simulink model "komparacija"  (R2020a)
settings: Solver=ode5  StartTime=0.0  StopTime=tfin  FixedStep=1e-3  RelTol=1e-3
values from neighbouring files (symbols this model uses):
  beta = S_upper_limit*w0/2    (= 0.06550194)    [komparacija_matlab.m]
  derivative_e_lower_limit = -7.8663    [komparacija_matlab.m]
  derivative_e_upper_limit = 7.8663    [komparacija_matlab.m]
  disturb_X = 0.2*Xe    (= 0.978133730754)    [komparacija_matlab.m]
  disturb_X_time = 5    [komparacija_matlab.m]
  F_lower_limit = 0    [komparacija_matlab.m]
  F_upper_limit = Fe + 1e-3*Fe    (= 3.21211951185)    [komparacija_matlab.m]
  F_upper_limit_PI = 1e-3*Fe    (= 0.00320891060125)    [komparacija_matlab.m]
  Fe = 3.20891060125344    (= 3.20891060125)    [komparacija_matlab.m]
  Fi = beta/5/w0    (= 0.02324)    [komparacija_matlab.m]
  K0_FLRT = w0    (= 0.5637)    [komparacija_matlab.m]
  K1 = 0.0300    (= 0.03)    [komparacija_matlab.m]
  K2 = 0.5000    (= 0.5)    [komparacija_matlab.m]
  Kc1 = 1/abs(freqresp((1+1/Ti1/s)*G_design,w1_design))    [komparacija_matlab.m]
  Ki = 0    [komparacija_matlab.m]
  mi0 = mie    (= 0.802227650313)    [komparacija_matlab.m]
  mi_max = 1    [komparacija_matlab.m]
  S_step1 = delta    (= 0)    [komparacija_matlab.m]
  S_step2 = delta    (= 0)    [komparacija_matlab.m]
  S_time_step1 = 20    [komparacija_matlab.m]
  S_time_step2 = 50    [komparacija_matlab.m]
  Se = 0.218662692463450    (= 0.218662692463)    [komparacija_matlab.m]
  SF = 10.0000    (= 10)    [komparacija_matlab.m]
  std_noise = 1e-5*Se    (= 2.18662692463e-06)    [komparacija_matlab.m]
  V = 4.0000    (= 4)    [komparacija_matlab.m]
  x10 = Xe    (= 4.89066865377)    [komparacija_matlab.m]
  x20 = Se    (= 0.218662692463)    [komparacija_matlab.m]
  Y = 0.5000    (= 0.5)    [komparacija_matlab.m]
undefined symbols (not defined in the file or in its folder): magnitude
libraries: fuzblock x1, cstblocks x1
settings Model: Creator=anaMceranic  LastModifiedBy=anaMceranic
settings DataIOCC: ReturnWorkspaceOutputs=off

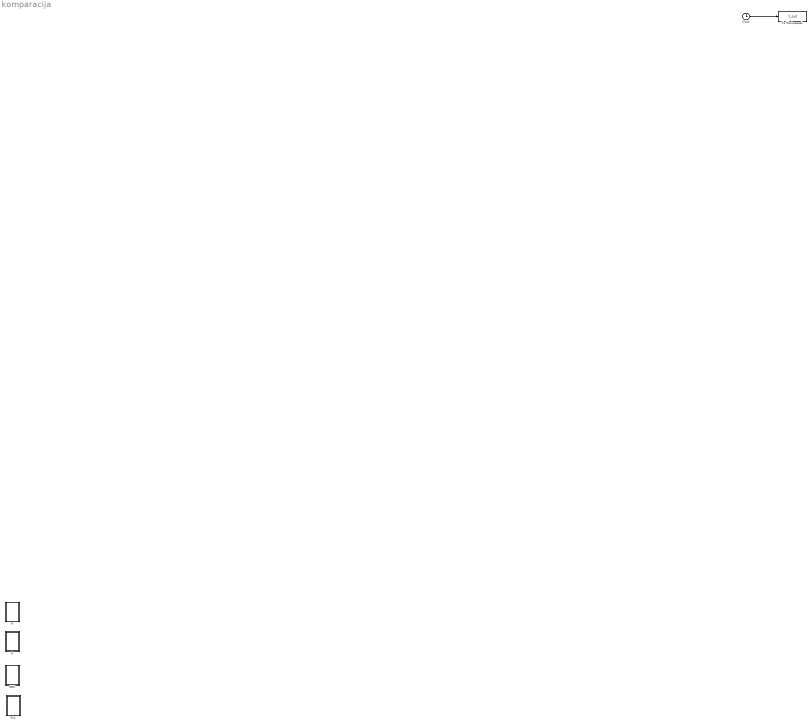
== system komparacija ==
  Clock : Clock
  FLC : Subsystem
  PI : Subsystem
  SMC : Subsystem
  To Workspace1 : ToWorkspace  VariableName=t_out  SampleTime=-1
  fl : Subsystem
  wires:
  Clock/1 -> To Workspace1/1

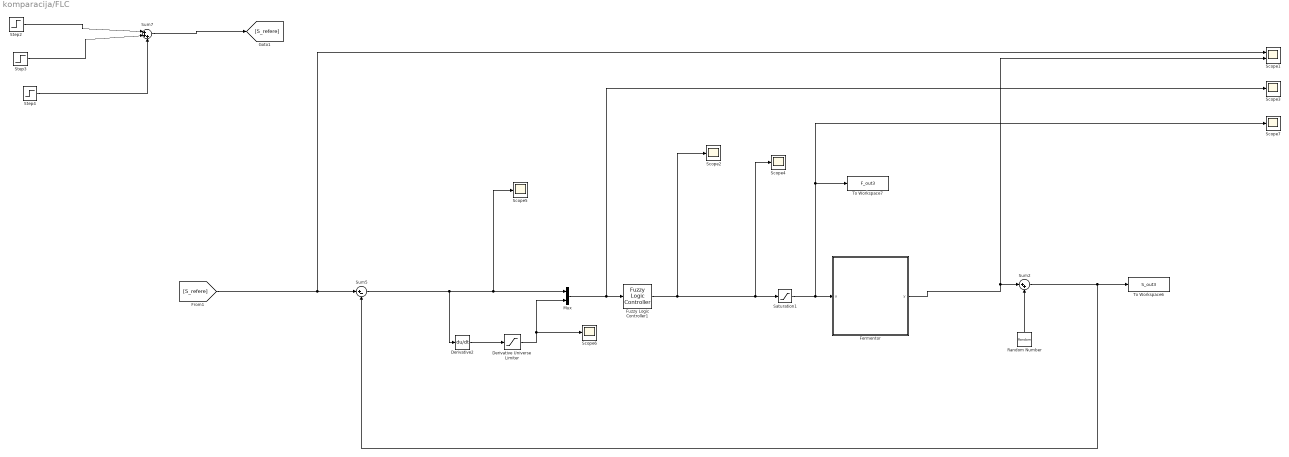
== system komparacija/FLC ==
  Derivative Universe Limiter : Saturate  UpperLimit=derivative_e_upper_limit  LowerLimit=derivative_e_lower_limit
  Derivative2 : Derivative
  Fermentor : Subsystem
  Fuzzy Logic Controller1 : fuzblock/Fuzzy Logic  Controller  FIS=FLC  OutputSampleNumber=101  DataType=double  FuzzifiedInputs=off  RuleFiringStrengths=off  RuleOutputs=off  AggregatedOutputs=off  SimulateUsing=Interpreted execution  OutOfRangeInputValueMessage=warning  NoRuleFiredMessage=warning  EmptyOutputFuzzySetMessage=warning
  Mux : Mux  Inputs=2
  Random Number : RandomNumber  Variance=std_noise  SampleTime=0.1
  Saturation1 : Saturate  UpperLimit=F_upper_limit  LowerLimit=F_lower_limit
  Scope1 : Scope  NumInputPorts=2
  Scope{2..7} (6 alike) : Scope
  Step2 : Step  Time=0  Before=Se  After=Se  SampleTime=0
  Step3 : Step  Time=S_time_step1  After=S_step1  SampleTime=0
  Step4 : Step  Time=S_time_step2  After=-S_step2  SampleTime=0
  Sum2 : Sum  Inputs=|++
  Sum5 : Sum  Inputs=|+-
  Sum7 : Sum  Inputs=|+++
  To Workspace6 : ToWorkspace  VariableName=S_out3  SampleTime=-1
  To Workspace7 : ToWorkspace  VariableName=F_out3  SampleTime=-1
  wires:
  Fuzzy Logic Controller1/1 -> Scope4/1, Saturation1/1, Scope2/1
  Sum5/1 -> Derivative2/1, Scope5/1, Mux/1
  [S_refere] -> Scope1/1, Sum5/1
  Fermentor/1(y) -> Scope1/2, Sum2/1
  Sum2/1 -> Sum5/2, To Workspace6/1
  Step2/1 -> Sum7/1
  Saturation1/1 -> Scope7/1, To Workspace7/1, Fermentor/1(u)
  Random Number/1 -> Sum2/2
  Derivative Universe Limiter/1 -> Scope6/1, Mux/2
  Mux/1 -> Fuzzy Logic Controller1/1, Scope3/1
  Step3/1 -> Sum7/2
  Sum7/1 -> [S_refere]
  Derivative2/1 -> Derivative Universe Limiter/1
  Step4/1 -> Sum7/3

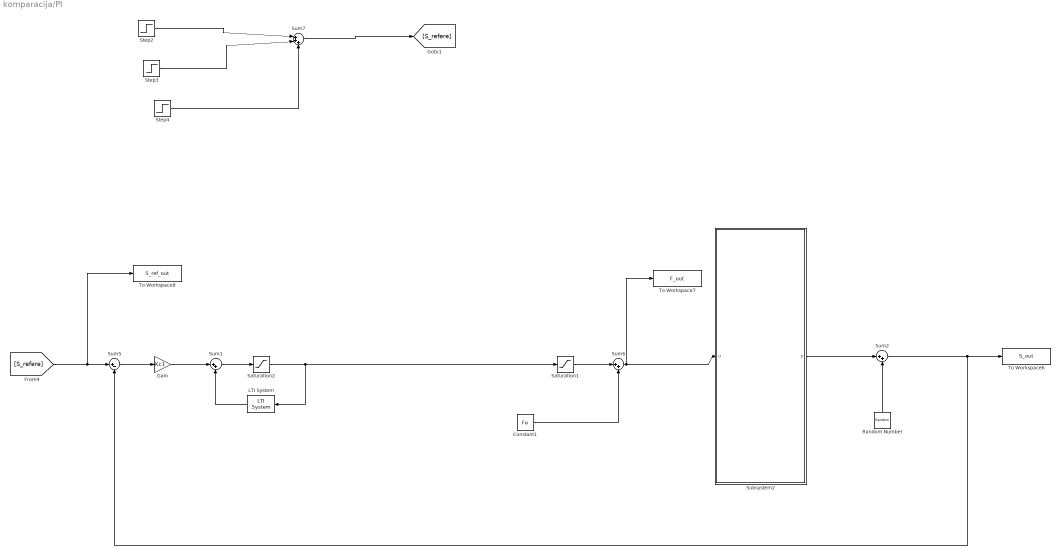
== system komparacija/PI ==
  Constant1 : Constant  Value=Fe
  Gain : Gain  Gain=Kc1
  LTI System : cstblocks/LTI System  sys=KPI_aw  IC=[]
  Random Number : RandomNumber  Variance=std_noise  SampleTime=0.1
  Saturation1 : Saturate  UpperLimit=F_upper_limit_PI  LowerLimit=F_lower_limit
  Saturation2 : Saturate  UpperLimit=F_upper_limit  LowerLimit=F_lower_limit
  Step2 : Step  Time=0  Before=Se  After=Se  SampleTime=0
  Step3 : Step  Time=S_time_step1  After=S_step1  SampleTime=0
  Step4 : Step  Time=S_time_step2  After=-S_step2  SampleTime=0
  Subsystem2 : Subsystem
  Sum1 : Sum  Inputs=|++
  Sum2 : Sum  Inputs=|++
  Sum5 : Sum  Inputs=|+-
  Sum6 : Sum  Inputs=|++
  Sum7 : Sum  Inputs=|+++
  To Workspace6 : ToWorkspace  VariableName=S_out  SampleTime=-1
  To Workspace7 : ToWorkspace  VariableName=F_out  SampleTime=-1
  To Workspace8 : ToWorkspace  VariableName=S_ref_out  SampleTime=-1
  wires:
  [S_refere] -> To Workspace8/1, Sum5/1
  Sum5/1 -> Gain/1
  Saturation2/1 -> Saturation1/1, LTI System/1
  Sum6/1 -> To Workspace7/1, Subsystem2/1(u)
  Sum1/1 -> Saturation2/1
  Sum7/1 -> [S_refere]
  Constant1/1 -> Sum6/2
  Subsystem2/1(y) -> Sum2/1
  Gain/1 -> Sum1/1
  Step2/1 -> Sum7/1
  Saturation1/1 -> Sum6/1
  Step4/1 -> Sum7/3
  Step3/1 -> Sum7/2
  Sum2/1 -> Sum5/2, To Workspace6/1
  Random Number/1 -> Sum2/2
  LTI System/1 -> Sum1/2

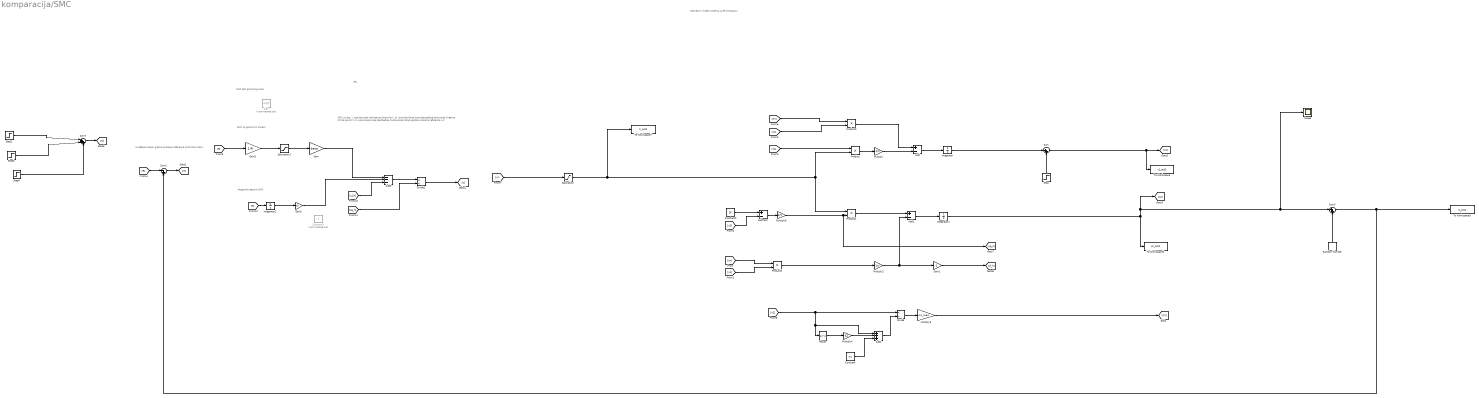
== system komparacija/SMC ==
  note: SMC bez graničnog sloja
  note: eFL
  note: integralno dejstvo SMC
  note: SMC skupa:
      | 1. poništavanje nelinearne dinamike
      | 2. a) upravljavljanje koje obezbeđuje dostizanje linearne klizne površi
      | 2. b) upravljanje koje obezbeđuje zavšavanje stanja greške praćenja reference u 0
  note: Nelinearni model sistema za fermentaciju
  note: SMC sa graničnim slojem
  note: Uvođenje stanja:
      | greška praćenja reference od strane izlaza
  Add : Sum  Inputs=+-
  Add1 : Sum  Inputs=+-
  Add2 : Sum  Inputs=+++
  Add3 : Sum  Inputs=---
  Constant : Constant  Value=K1
  Constant1 : Constant  Commented=on  Value=0
  Constant2 : Constant  Value=SF
  Divide : Product  Inputs=*/
  Divide1 : Product  Inputs=*/
  Gain : Gain  Gain=beta
  Gain1 : Gain  Gain=-1
  Gain2 : Gain  Gain=Ki
  Gain3 : Gain  Gain=1/Fi
  Integrator : Integrator  InitialCondition=x10
  Integrator1 : Integrator  InitialCondition=x20
  Integrator2 : Integrator
  Multiply : Gain  Gain=1/V
  Multiply2 : Gain  Gain=1/Y
  Multiply3 : Gain  Gain=mi_max
  Multiply4 : Gain  Gain=K2
  Multiply6 : Gain  Gain=1/V
  Power : Math  Operator=magnitude^2  SaturateOnIntegerOverflow=on
  Product{,1..3} (4 alike) : Product
  Random Number : RandomNumber  Variance=std_noise  SampleTime=0.1
  Saturation : Saturate  UpperLimit=F_upper_limit  LowerLimit=F_lower_limit
  Saturation1 : Saturate
  Scope : Scope
  Sign : Signum  Commented=on
  Step : Step  Time=disturb_X_time  After=disturb_X  SampleTime=0
  Step2 : Step  Time=0  Before=Se  After=Se  SampleTime=0
  Step3 : Step  Time=S_time_step1  After=S_step1  SampleTime=0
  Step4 : Step  Time=S_time_step2  After=-S_step2  SampleTime=0
  Subtract : Sum  Inputs=+-
  Sum : Sum  Inputs=|++
  Sum2 : Sum  Inputs=|-+
  Sum3 : Sum  Inputs=|++
  Sum7 : Sum  Inputs=|+++
  To Workspace : ToWorkspace  VariableName=x1_out2  SampleTime=-1
  To Workspace2 : ToWorkspace  VariableName=x2_out2  SampleTime=-1
  To Workspace3 : ToWorkspace  VariableName=S_out2  SampleTime=-1
  To Workspace7 : ToWorkspace  VariableName=F_out2  SampleTime=-1
  wires:
  Step/1 -> Sum/2
  Integrator/1 -> Sum/1
  [mi] -> Product3/1
  [mi] -> Product2/1
  [e] -> Gain3/1
  Product3/1 -> Add/1
  Subtract/1 -> Multiply6/1
  Sum3/1 -> Sum2/2, To Workspace3/1
  Multiply3/1 -> [mi]
  Saturation/1 -> To Workspace7/1, Product1/1, Product/2
  Gain3/1 -> Saturation1/1
  Saturation1/1 -> Gain/1
  Add3/1 -> Divide1/1
  Constant2/1 -> Subtract/1
  [Lf_h] -> Add3/3
  Integrator1/1 -> Scope/1, Sum3/1, [x2], To Workspace2/1
  Multiply2/1 -> Gain1/1, Add1/2
  Constant/1 -> Add2/3
  Product2/1 -> Multiply2/1
  [x1] -> Product/1
  Sum7/1 -> [R]
  Multiply4/1 -> Add2/2
  Product/1 -> Multiply/1
  Step3/1 -> Sum7/2
  Add2/1 -> Divide/2
  [x2] -> Subtract/2
  [u] -> Saturation/1
  Gain/1 -> Add3/1
  Add/1 -> Integrator/1
  Step2/1 -> Sum7/1
  Integrator2/1 -> Gain2/1
  Multiply6/1 -> [Lg_h], Product1/2
  Divide/1 -> Multiply3/1
  Gain2/1 -> Add3/2
  Gain1/1 -> [Lf_h]
  [x1] -> Product3/2
  [e] -> Integrator2/1
  [R] -> Sum2/1
  Sum2/1 -> [e]
  [Lg_h] -> Divide1/2
  Random Number/1 -> Sum3/2
  Divide1/1 -> [u]
  Product1/1 -> Add1/1
  [x1] -> Product2/2
  Add1/1 -> Integrator1/1
  Sum/1 -> [x1], To Workspace/1
  Multiply/1 -> Add/2
  Step4/1 -> Sum7/3
  [x2] -> Power/1, Add2/1, Divide/1
  Power/1 -> Multiply4/1

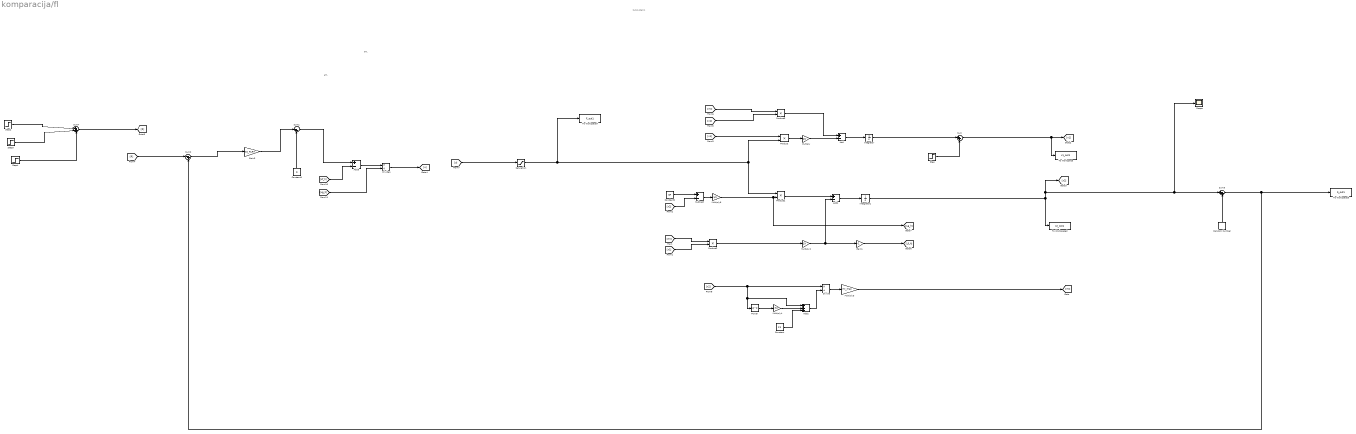
== system komparacija/fl ==
  note: eFL
  note: Subsystem1
  note: eFL
  Add : Sum  Inputs=+-
  Add1 : Sum  Inputs=+-
  Add2 : Sum  Inputs=+++
  Add3 : Sum  Inputs=+-
  Constant : Constant  Value=K1
  Constant1 : Constant  Value=0
  Constant2 : Constant  Value=SF
  Divide : Product  Inputs=*/
  Divide1 : Product  Inputs=*/
  Gain1 : Gain  Gain=-1
  Gain3 : Gain  Gain=K0_FLRT
  Integrator : Integrator  InitialCondition=x10
  Integrator1 : Integrator  InitialCondition=x20
  Multiply : Gain  Gain=1/V
  Multiply2 : Gain  Gain=1/Y
  Multiply3 : Gain  Gain=mi_max
  Multiply4 : Gain  Gain=K2
  Multiply6 : Gain  Gain=1/V
  Power : Math  Operator=magnitude^2  SaturateOnIntegerOverflow=on
  Product{,1..3} (4 alike) : Product
  Random Number : RandomNumber  Variance=std_noise  SampleTime=0.1
  Saturation : Saturate  UpperLimit=F_upper_limit  LowerLimit=F_lower_limit
  Scope : Scope
  Step : Step  Time=5  After=disturb_X  SampleTime=0
  Step2 : Step  Time=0  Before=Se  After=Se  SampleTime=0
  Step3 : Step  Time=S_time_step1  After=S_step1  SampleTime=0
  Step4 : Step  Time=S_time_step2  After=-S_step2  SampleTime=0
  Subtract : Sum  Inputs=+-
  Sum : Sum  Inputs=|++
  Sum1 : Sum  Inputs=|--
  Sum2 : Sum  Inputs=|-+
  Sum3 : Sum  Inputs=|++
  Sum7 : Sum  Inputs=|+++
  To Workspace : ToWorkspace  VariableName=x1_out1  SampleTime=-1
  To Workspace2 : ToWorkspace  VariableName=x2_out1  SampleTime=-1
  To Workspace3 : ToWorkspace  VariableName=S_out1  SampleTime=-1
  To Workspace7 : ToWorkspace  VariableName=F_out1  SampleTime=-1
  wires:
  Saturation/1 -> To Workspace7/1, Product1/1, Product/2
  [x2] -> Power/1, Add2/1, Divide/1
  [x2] -> Subtract/2
  Product3/1 -> Add/1
  [mi] -> Product2/1
  Integrator1/1 -> Scope/1, Sum3/1, [x2], To Workspace2/1
  Sum3/1 -> Sum2/2, To Workspace3/1
  Constant1/1 -> Sum1/2
  Step4/1 -> Sum7/3
  Subtract/1 -> Multiply6/1
  [x1] -> Product/1
  Sum7/1 -> [R]
  Step/1 -> Sum/2
  Multiply4/1 -> Add2/2
  [x1] -> Product3/2
  Gain3/1 -> Sum1/1
  Add3/1 -> Divide1/1
  Sum1/1 -> Add3/1
  Multiply3/1 -> [mi]
  [R] -> Sum2/1
  Sum2/1 -> Gain3/1
  Add2/1 -> Divide/2
  Product/1 -> Multiply/1
  Add1/1 -> Integrator1/1
  [u] -> Saturation/1
  Constant/1 -> Add2/3
  Multiply/1 -> Add/2
  Product1/1 -> Add1/1
  Power/1 -> Multiply4/1
  Multiply2/1 -> Gain1/1, Add1/2
  Multiply6/1 -> [Lg_h], Product1/2
  Divide1/1 -> [u]
  [Lf_h] -> Add3/2
  Divide/1 -> Multiply3/1
  Gain1/1 -> [Lf_h]
  Add/1 -> Integrator/1
  Integrator/1 -> Sum/1
  Constant2/1 -> Subtract/1
  Product2/1 -> Multiply2/1
  Sum/1 -> [x1], To Workspace/1
  Step3/1 -> Sum7/2
  [x1] -> Product2/2
  [Lg_h] -> Divide1/2
  [mi] -> Product3/1
  Random Number/1 -> Sum3/2
  Step2/1 -> Sum7/1

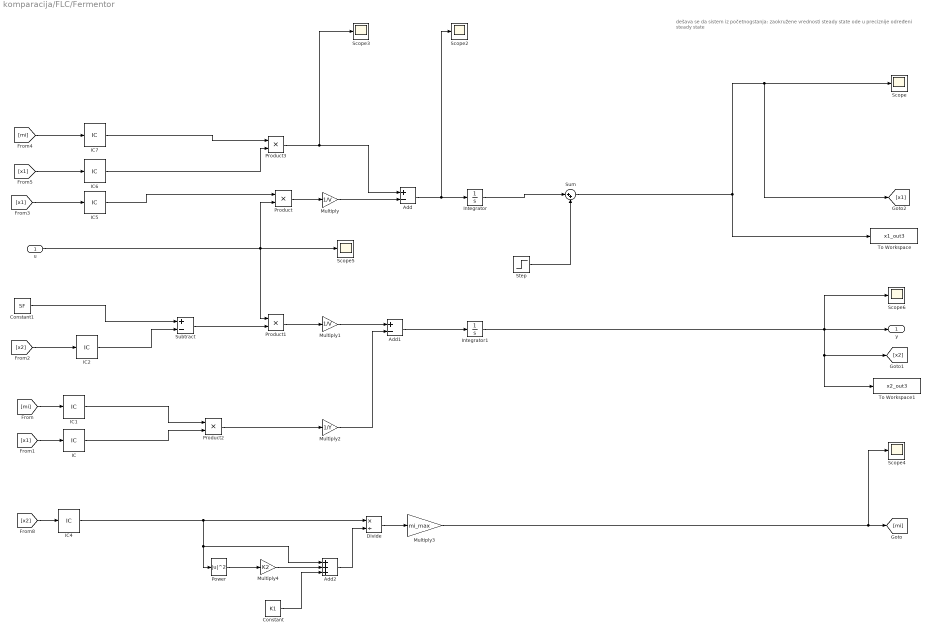
== system komparacija/FLC/Fermentor ==
  note: dešava se da sistem iz početnogstanja: zaokružene vrednosti steady state
      | ode u preciznije određeni steady state
  u : Inport
  Add : Sum  Inputs=+-
  Add1 : Sum  Inputs=+-
  Add2 : Sum  Inputs=+++
  Constant : Constant  Value=K1
  Constant1 : Constant  Value=SF
  Divide : Product  Inputs=*/
  IC : InitialCondition  Value=x10
  IC1 : InitialCondition  Value=mi0
  IC2 : InitialCondition  Value=x20
  IC4 : InitialCondition  Value=x20
  IC5 : InitialCondition  Value=x10
  IC6 : InitialCondition  Value=x10
  IC7 : InitialCondition  Value=mi0
  Integrator : Integrator  InitialCondition=x10
  Integrator1 : Integrator  InitialCondition=x20
  Multiply : Gain  Gain=1/V
  Multiply1 : Gain  Gain=1/V
  Multiply2 : Gain  Gain=1/Y
  Multiply3 : Gain  Gain=mi_max
  Multiply4 : Gain  Gain=K2
  Power : Math  Operator=magnitude^2  SaturateOnIntegerOverflow=on
  Product{,1..3} (4 alike) : Product
  Scope{,2..6} (6 alike) : Scope
  Step : Step  Time=disturb_X_time  After=disturb_X  SampleTime=0
  Subtract : Sum  Inputs=+-
  Sum : Sum  Inputs=|++
  To Workspace : ToWorkspace  VariableName=x1_out3  SampleTime=-1
  To Workspace1 : ToWorkspace  VariableName=x2_out3  SampleTime=-1
  y : Outport
  wires:
  [x1] -> IC/1
  Product2/1 -> Multiply2/1
  Multiply/1 -> Add/2
  Add2/1 -> Divide/2
  Constant/1 -> Add2/3
  [x1] -> IC6/1
  Multiply4/1 -> Add2/2
  [mi] -> IC1/1
  Power/1 -> Multiply4/1
  [x2] -> IC2/1
  Add1/1 -> Integrator1/1
  Multiply2/1 -> Add1/2
  Divide/1 -> Multiply3/1
  Product3/1 -> Scope3/1, Add/1
  u/1 -> Product/2, Product1/1, Scope5/1
  [x1] -> IC5/1
  Multiply1/1 -> Add1/1
  Product1/1 -> Multiply1/1
  Subtract/1 -> Product1/2
  [x2] -> IC4/1
  Add/1 -> Scope2/1, Integrator/1
  Product/1 -> Multiply/1
  [mi] -> IC7/1
  Multiply3/1 -> [mi], Scope4/1
  Integrator1/1 -> Scope6/1, To Workspace1/1, [x2], y/1
  IC/1 -> Product2/2
  IC1/1 -> Product2/1
  IC2/1 -> Subtract/2
  Constant1/1 -> Subtract/1
  IC4/1 -> Divide/1, Add2/1, Power/1
  IC5/1 -> Product/1
  IC6/1 -> Product3/2
  IC7/1 -> Product3/1
  Sum/1 -> To Workspace/1, Scope/1, [x1]
  Step/1 -> Sum/2
  Integrator/1 -> Sum/1

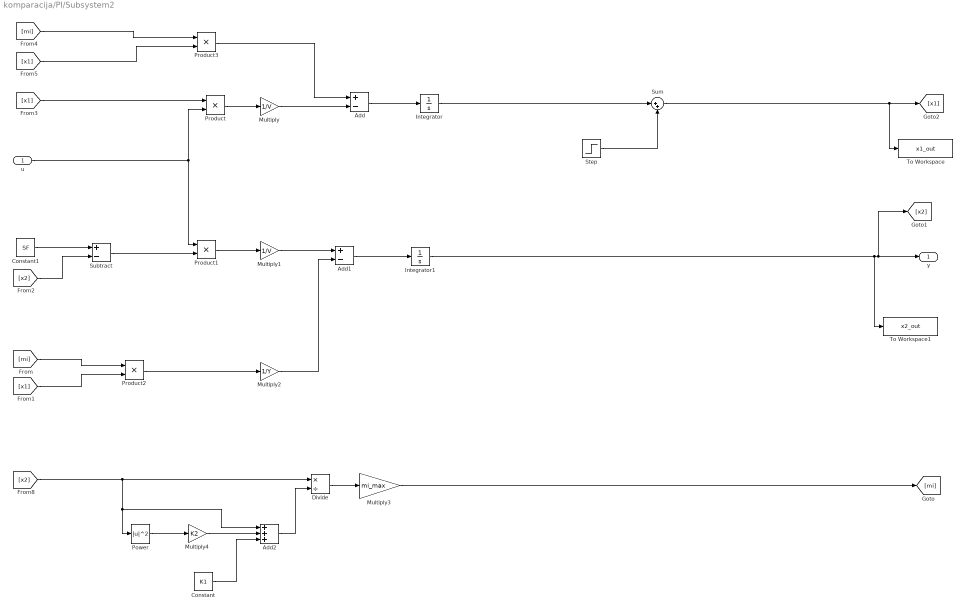
== system komparacija/PI/Subsystem2 ==
  u : Inport
  Add : Sum  Inputs=+-
  Add1 : Sum  Inputs=+-
  Add2 : Sum  Inputs=+++
  Constant : Constant  Value=K1
  Constant1 : Constant  Value=SF
  Divide : Product  Inputs=*/
  Integrator : Integrator  InitialCondition=x10
  Integrator1 : Integrator  InitialCondition=x20
  Multiply : Gain  Gain=1/V
  Multiply1 : Gain  Gain=1/V
  Multiply2 : Gain  Gain=1/Y
  Multiply3 : Gain  Gain=mi_max
  Multiply4 : Gain  Gain=K2
  Power : Math  Operator=magnitude^2  SaturateOnIntegerOverflow=on
  Product{,1..3} (4 alike) : Product
  Step : Step  Time=5  After=disturb_X  SampleTime=0
  Subtract : Sum  Inputs=+-
  Sum : Sum  Inputs=|++
  To Workspace : ToWorkspace  VariableName=x1_out  SampleTime=-1
  To Workspace1 : ToWorkspace  VariableName=x2_out  SampleTime=-1
  y : Outport
  wires:
  [x1] -> Product2/2
  Product2/1 -> Multiply2/1
  Multiply/1 -> Add/2
  Add2/1 -> Divide/2
  Constant/1 -> Add2/3
  [x1] -> Product3/2
  Multiply4/1 -> Add2/2
  [mi] -> Product2/1
  Multiply3/1 -> [mi]
  Power/1 -> Multiply4/1
  Constant1/1 -> Subtract/1
  [x2] -> Subtract/2
  Add1/1 -> Integrator1/1
  Multiply2/1 -> Add1/2
  Integrator1/1 -> [x2], y/1, To Workspace1/1
  Divide/1 -> Multiply3/1
  Product3/1 -> Add/1
  u/1 -> Product1/1, Product/2
  [x1] -> Product/1
  Multiply1/1 -> Add1/1
  Product1/1 -> Multiply1/1
  Subtract/1 -> Product1/2
  [x2] -> Divide/1, Add2/1, Power/1
  Add/1 -> Integrator/1
  Product/1 -> Multiply/1
  [mi] -> Product3/1
  Integrator/1 -> Sum/1
  Sum/1 -> To Workspace/1, [x1]
  Step/1 -> Sum/2
